simulink library "Tools"  (R2012b)
settings: Solver=ode45  StartTime=0.0  StopTime=10.0  RelTol=1e-3
libraries: simulink x1
settings Model: Creator=h3now  LastModifiedBy=h3now

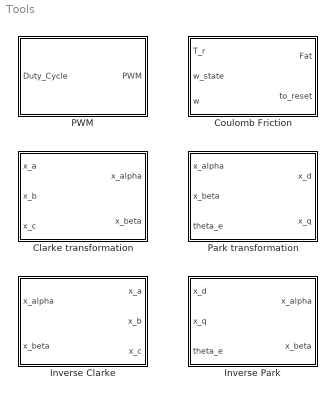
== system Tools ==
  Clarke transformation : Subsystem
  Coulomb Friction : Subsystem  mask(Modelo de atrito de Coulomb){F_stick=0.01, F_slip=0.005}
      mask prompts: F_stick "Torque máxima de atrito estático [N.m]"; F_slip "Torque de atrito dinâmico [N.m]"
      mask help:
      | Entradas
      | - T_r: Torque líquido que está sendo aplicado no rotor[N.m]
      | - w_state: Essa entrada deve ser conectada ao "state port" do integrador cuja saída é a velocidade angular do rotor para não gerar loops algébricos
      | - w: Velocidade angular do rotor [unidade não importa]
      |
      | Saídas
      | - Fat: Torque de atrito [N.m]
      | - to_reset: Essa saída deve ser conectada ao reset do integrador cuja saída é a velocidade angular do rotor
  Inverse Clarke : Subsystem
  Inverse Park : Subsystem
  PWM : Subsystem  StartFcn=|  mask{f=20000}
      | T_PWM = get_param(gcb,'f');                                             
      | T_PWM = 1./str2double(T_PWM);                                           
      | T_solver = get_param(bdroot,'FixedStep');                               
      | T_solver = str2double(T_solver);                                        
      | if T_solver > 0.5*T_PWM                                                 
      |    %error('Solver step size must be smaller than 10% of the PWM period')
      | end
      mask prompts: f "PWM Frequency [Hz}"
      mask help:
      | Simula o funcionamento de um PWM.
      |
      | Duty_Cycle = Sinal que varia entre 0 e 1 e define o duty cycle do PWM.
  "Park transformation " : Subsystem

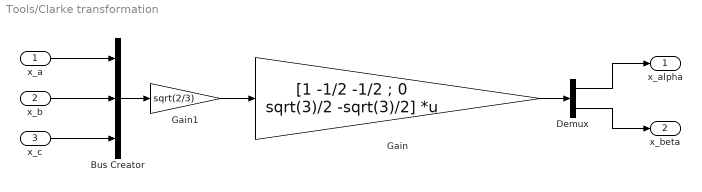
== system Tools/Clarke transformation ==
  x_a : Inport
  x_b : Inport  Port=2
  x_c : Inport  Port=3
  Bus Creator : BusCreator  Inputs=3
  Demux : Demux  Outputs=2
  Gain : Gain  Gain=[1 -1/2 -1/2 ; 0 sqrt(3)/2 -sqrt(3)/2]  Multiplication=Matrix(K*u)
  Gain1 : Gain  Gain=sqrt(2/3)
  x_alpha : Outport
  x_beta : Outport  Port=2
  wires:
  Demux/1 -> x_alpha/1
  Bus Creator/1 -> Gain1/1
  Demux/2 -> x_beta/1
  Gain/1 -> Demux/1
  x_a/1 -> Bus Creator/1
  x_c/1 -> Bus Creator/3
  x_b/1 -> Bus Creator/2
  Gain1/1 -> Gain/1

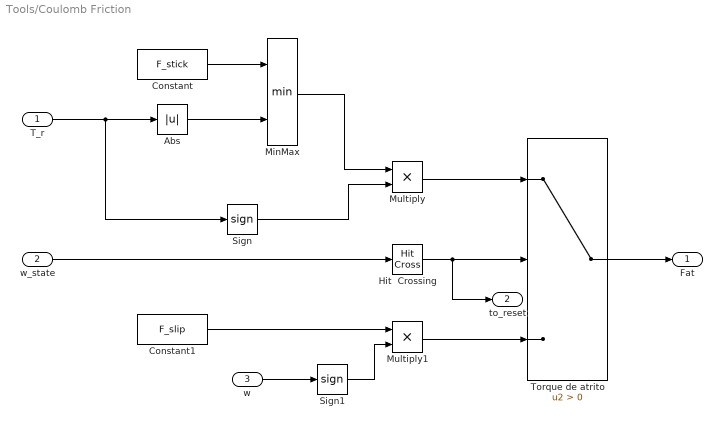
== system Tools/Coulomb Friction ==
  T_r : Inport
  w_state : Inport  Port=2
  w : Inport  Port=3
  Abs : Abs
  Constant : Constant  Value=F_stick
  Constant1 : Constant  Value=F_slip
  Hit  Crossing : HitCross
  MinMax : MinMax  Inputs=2
  Multiply : Product  Inputs=**
  Multiply1 : Product  Inputs=**
  Sign : Signum
  Sign1 : Signum
  Torque de atrito : Switch  Criteria=u2 > Threshold
  Fat : Outport
  to_reset : Outport  Port=2
  wires:
  Multiply/1 -> Torque de atrito/1
  Sign1/1 -> Multiply1/2
  MinMax/1 -> Multiply/1
  Abs/1 -> MinMax/2
  T_r/1 -> Abs/1, Sign/1
  Constant1/1 -> Multiply1/1
  Multiply1/1 -> Torque de atrito/3
  w_state/1 -> Hit  Crossing/1
  Hit  Crossing/1 -> Torque de atrito/2, to_reset/1
  Sign/1 -> Multiply/2
  w/1 -> Sign1/1
  Torque de atrito/1 -> Fat/1
  Constant/1 -> MinMax/1

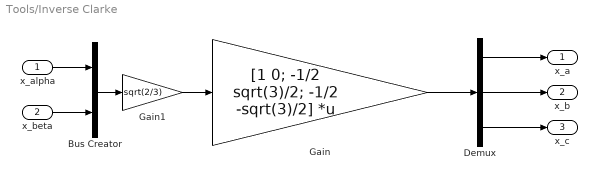
== system Tools/Inverse Clarke ==
  x_alpha : Inport
  x_beta : Inport  Port=2
  Bus Creator : BusCreator  Inputs=2
  Demux : Demux  Outputs=3
  Gain : Gain  Gain=[1 0; -1/2 sqrt(3)/2; -1/2 -sqrt(3)/2]  Multiplication=Matrix(K*u)
  Gain1 : Gain  Gain=sqrt(2/3)
  x_a : Outport
  x_b : Outport  Port=2
  x_c : Outport  Port=3
  wires:
  Bus Creator/1 -> Gain1/1
  Gain/1 -> Demux/1
  Demux/1 -> x_a/1
  Demux/2 -> x_b/1
  Demux/3 -> x_c/1
  x_beta/1 -> Bus Creator/2
  x_alpha/1 -> Bus Creator/1
  Gain1/1 -> Gain/1

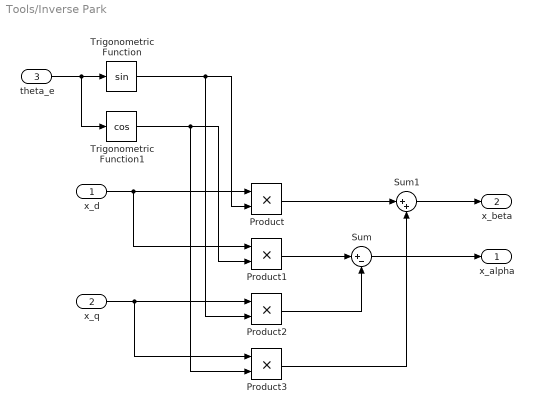
== system Tools/Inverse Park ==
  x_d : Inport
  x_q : Inport  Port=2
  theta_e : Inport  Port=3
  Product{,1..3} (4 alike) : Product  RndMeth=Zero
  Sum : Sum  Inputs=|+-
  Sum1 : Sum  Inputs=|++
  Trigonometric Function : Trigonometry  OutputSignalType=real
  Trigonometric Function1 : Trigonometry  Operator=cos  OutputSignalType=real
  "x_alpha " : Outport
  x_beta : Outport  Port=2
  wires:
  Product/1 -> Sum1/1
  Sum1/1 -> x_beta/1
  theta_e/1 -> Trigonometric Function1/1, Trigonometric Function/1
  x_d/1 -> Product/1, Product1/1
  Sum/1 -> "x_alpha "/1
  Trigonometric Function/1 -> Product2/2, Product/2
  Product3/1 -> Sum1/2
  Product2/1 -> Sum/2
  Trigonometric Function1/1 -> Product3/2, Product1/2
  x_q/1 -> Product3/1, Product2/1
  Product1/1 -> Sum/1

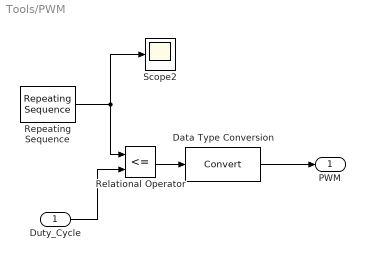
== system Tools/PWM ==
  Duty_Cycle : Inport
  Data Type Conversion : DataTypeConversion
  Relational Operator : RelationalOperator  Operator=<=  OutDataTypeStr=boolean
  Repeating Sequence : simulink/Sources/Repeating Sequence  rep_seq_t=[0 1/f]  rep_seq_y=[0 1]
  Scope2 : Scope
      settings: YMin=0.294  YMax=0.301
  PWM : Outport
  wires:
  Relational Operator/1 -> Data Type Conversion/1
  Data Type Conversion/1 -> PWM/1
  Repeating Sequence/1 -> Relational Operator/1, Scope2/1
  Duty_Cycle/1 -> Relational Operator/2

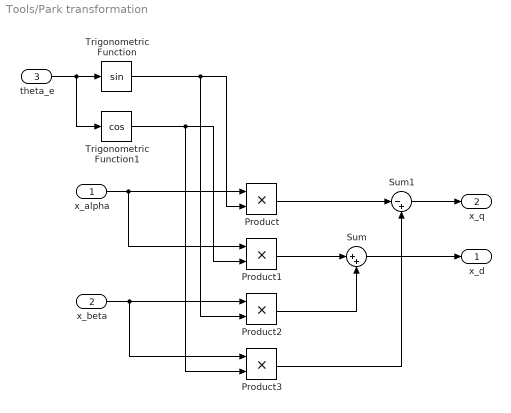
== system Tools/Park transformation  ==
  x_alpha : Inport
  x_beta : Inport  Port=2
  theta_e : Inport  Port=3
  Product{,1..3} (4 alike) : Product  RndMeth=Zero
  Sum : Sum  Inputs=|++
  Sum1 : Sum  Inputs=|-+
  Trigonometric Function : Trigonometry  OutputSignalType=real
  Trigonometric Function1 : Trigonometry  Operator=cos  OutputSignalType=real
  x_d : Outport
  x_q : Outport  Port=2
  wires:
  theta_e/1 -> Trigonometric Function1/1, Trigonometric Function/1
  x_alpha/1 -> Product/1, Product1/1
  x_beta/1 -> Product3/1, Product2/1
  Trigonometric Function/1 -> Product2/2, Product/2
  Trigonometric Function1/1 -> Product3/2, Product1/2
  Product1/1 -> Sum/1
  Product2/1 -> Sum/2
  Sum/1 -> x_d/1
  Product/1 -> Sum1/1
  Product3/1 -> Sum1/2
  Sum1/1 -> x_q/1
